simulink model "SegWay"  (R2019b)
settings: Solver=VariableStepAuto  StartTime=0.0  StopTime=2  RelTol=1e-3
values from neighbouring files (symbols this model uses):
  a21 = (m_t^2*g*r*l^2)/x_1    (= -2.65744560529)    [Untitled.m]    (also in main.m = -8.63813922358)
  a22 = (2*k_m*k_e*(m_t*l*r + m_t*l^2 + J_t))/(R*x_1)    (= -2.29592930526)    [Untitled.m]    (also in main.m = -7.58795528199)
  a31 = (-m_t*g*l*(m_t*r^2 + 2*m_k*r^2 + 2*J_k + 2*J))/x_1    (= 97.5739413998)    [Untitled.m]    (also in main.m = 82.5552904929)
  a32 = (-2*k_m*k_e*(m_t*l*r + m_t*r^2 + 2*m_k*r^2 + 2*J_k))/(R*x_1)    (= 15.1379836425)    [Untitled.m]    (also in main.m = 2.73343418736)
  b2 = (-2*k_m*(m_t*l*r + m_t*l^2 + J_t))/(R*x_1)    (= 7.91699760433)    [Untitled.m]    (also in main.m = 26.1653630413)
  b3 = (2*k_m*(m_t*l*r + m_t*r^2 + 2*m_k*r^2 + 2*J_k))/(R*x_1)    (= -52.1999435948)    [Untitled.m]    (also in main.m = -9.42563512882)
  k_1 = K(1,1)    [Untitled.m]    (also in main.m)
  k_2 = K(2,1)    [Untitled.m]    (also in main.m)
  k_3 = K(3,1)    [Untitled.m]    (also in main.m)
  Um = 6    [Untitled.m]    (also in main.m = 8)
settings Model: Creator=Ivan  LastModifiedBy=Ivan

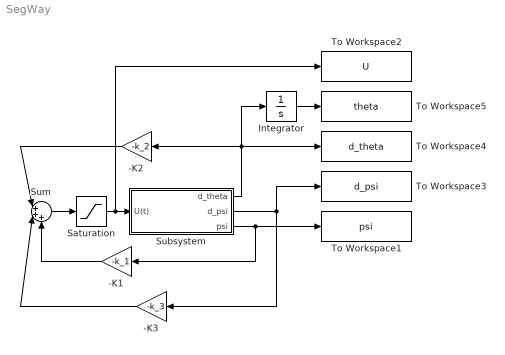
== system SegWay ==
  "-K1 " : Gain  Gain=-k_1
  -K2 : Gain  Gain=-k_2
  "-K3 " : Gain  Gain=-k_3
  Integrator : Integrator
  Saturation : Saturate  UpperLimit=Um  LowerLimit=-Um
  Subsystem : Subsystem
  Sum : Sum  Inputs=|+++
  To Workspace1 : ToWorkspace  VariableName=psi  SaveFormat=Timeseries  SampleTime=-1
  To Workspace2 : ToWorkspace  VariableName=U  SaveFormat=Timeseries  SampleTime=-1
  To Workspace3 : ToWorkspace  VariableName=d_psi  SaveFormat=Timeseries  SampleTime=-1
  To Workspace4 : ToWorkspace  VariableName=d_theta  SaveFormat=Timeseries  SampleTime=-1
  To Workspace5 : ToWorkspace  VariableName=theta  SaveFormat=Timeseries  SampleTime=-1
  wires:
  Saturation/1 -> To Workspace2/1, Subsystem/1(U(t))
  Sum/1 -> Saturation/1
  Subsystem/1("d_theta ") -> Integrator/1, -K2/1, To Workspace4/1
  -K2/1 -> Sum/1
  Subsystem/3(psi) -> To Workspace1/1, "-K1 "/1
  "-K1 "/1 -> Sum/3
  Subsystem/2("d_psi ") -> To Workspace3/1, "-K3 "/1
  "-K3 "/1 -> Sum/2
  Integrator/1 -> To Workspace5/1

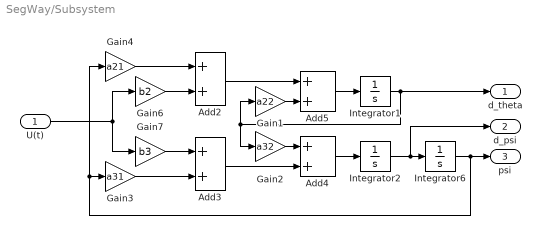
== system SegWay/Subsystem ==
  U(t) : Inport
  Add{2..5} (4 alike) : Sum
  Gain1 : Gain  Gain=a22
  Gain2 : Gain  Gain=a32
  Gain3 : Gain  Gain=a31
  Gain4 : Gain  Gain=a21
  Gain6 : Gain  Gain=b2
  Gain7 : Gain  Gain=b3
  Integrator1 : Integrator
  Integrator2 : Integrator
  Integrator6 : Integrator  InitialCondition=pi/12
  "d_theta " : Outport  Tag=D_Theta
  "d_psi " : Outport  Port=2
  psi : Outport  Port=3
  wires:
  U(t)/1 -> Gain7/1, Gain6/1
  Gain6/1 -> Add2/2
  Gain7/1 -> Add3/1
  Add3/1 -> Add4/2
  Add2/1 -> Add5/1
  Gain1/1 -> Add5/2
  Gain2/1 -> Add4/1
  Add5/1 -> Integrator1/1
  Add4/1 -> Integrator2/1
  Integrator1/1 -> "d_theta "/1, Gain2/1, Gain1/1
  Integrator2/1 -> "d_psi "/1, Integrator6/1
  Integrator6/1 -> Gain4/1, Gain3/1, psi/1
  Gain4/1 -> Add2/1
  Gain3/1 -> Add3/2
